simulink model "prob6"  (Simulink 7.6)
settings: Solver=ode45  StartTime=0.0  StopTime=1  RelTol=1e-3
settings Model: Creator=Dan  LastModifiedBy=Dan

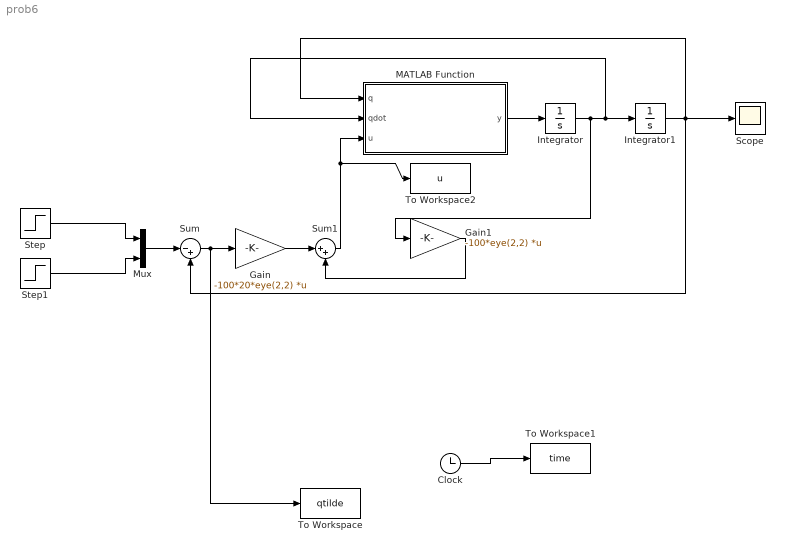
== system prob6 ==
  Clock : Clock
      settings: Decimation=10
  Gain : Gain  Gain=-100*20*eye(2,2)  Multiplication=Matrix(K*u)
  Gain1 : Gain  Gain=-100*eye(2,2)  Multiplication=Matrix(K*u)
  Integrator : Integrator  InitialCondition=[0;0];
  Integrator1 : Integrator  InitialCondition=[0;0];
  MATLAB Function : Stateflow chart  TreatAsAtomicUnit=on
  Mux : Mux  Inputs=2
  Scope : Scope
  Step : Step  Time=0  SampleTime=0
  Step1 : Step  Time=0  After=2  SampleTime=0
  Sum : Sum  Inputs=|-+
  Sum1 : Sum  Inputs=|++
  To Workspace : ToWorkspace  VariableName=qtilde  SampleTime=-1  SaveFormat=Array
  To Workspace1 : ToWorkspace  VariableName=time  SampleTime=-1  SaveFormat=Array
  To Workspace2 : ToWorkspace  VariableName=u  SampleTime=-1  SaveFormat=Array
  wires:
  MATLAB Function/1(y) -> Integrator/1
  Integrator/1 -> Integrator1/1, MATLAB Function/2(qdot), Gain1/1
  Step/1 -> Mux/1
  Step1/1 -> Mux/2
  Mux/1 -> Sum/1
  Integrator1/1 -> Sum/2, MATLAB Function/1(q), Scope/1
  Sum/1 -> Gain/1, To Workspace/1
  Gain/1 -> Sum1/1
  Gain1/1 -> Sum1/2
  Sum1/1 -> MATLAB Function/3(u), To Workspace2/1
  Clock/1 -> To Workspace1/1

== matlab function MATLAB Function ==
  data: q input double; y output double; qdot input double; u input double
function y = fcn(q,qdot,u)
%#codegen

q1=q(1);
q2=q(2);
qdot1=qdot(1);
qdot2=qdot(2);

M1=1;
L1=1;
Me=2;
de=30*pi/180;
I1=0.12;
Lc1=0.5;
Ie=0.25;
Lce=0.6;

a1=I1+M1*Lc1^2+Ie+Me*Lce^2+Me*L1^2;
a2=Ie+Me*Lce^2;
a3=Me*L1*Lce*cos(de);
a4=Me*L1*Lce*sin(de);

H11=a1+2*a3*cos(q2)+2*a4*sin(q2);
H12=a2+a3*cos(q2)+a4*sin(q2);
H21=H12;
H22=a2;
h=a3*sin(q2)-a4*cos(q2);



H=[H11 H12; H21 H22];
C=[-h*qdot2 -h*(qdot1+qdot2); h*qdot1 0];

y = -inv(H)*C*qdot+inv(H)*u;
